simulink model "receiving_app2"  (R2022b)
settings: Solver=FixedStepAuto  StartTime=0.0  StopTime=inf  RelTol=1e-3
libraries: androidcommunicationlib x3, androiduilib x3, androidaudiovideolib x1
settings Model: Creator=Akshat  LastModifiedBy=Akshat
settings OptimizationCC: EnhancedBackFolding=on  PassReuseOutputArgsAs=Individual arguments  ZeroExternalMemoryAtStartup=off  ZeroInternalMemoryAtStartup=off  MaxStackSize=64  OptimizeBlockOrder=speed  DifferentSizesBufferReuse=on  OptimizationCustomize=off  EfficientTunableParamExpr=on
settings DebuggingCC: ParameterTunabilityLossMsg=error
settings HardwareCC: ProdBitPerPointer=32  ProdBitPerSizeT=32  ProdBitPerPtrDiffT=32  ProdLargestAtomicInteger=Long  ProdLargestAtomicFloat=Double  ProdWordSize=32  ProdHWDeviceType=ARM Compatible->ARM Cortex  UseEmbeddedCoderFeatures=off
settings SFSimCC: MATLABDynamicMemAlloc=off
settings RTWCC: Description=Embedded Coder  SystemTargetFile=ert.tlc  HardwareBoard=Android Device  TLCOptions="-aInlineSetEventsForThisBaseRateFcn=TLC_FALSE -aSuppressMultiTaskScheduler=TLC_FALSE  -aRateBasedStepFcn=0"  TemplateMakefile=ert_default_tmf  RTWVerbose=off  Toolchain=Android SDK/NDK Tools
settings CodeAppCC: ForceParamTrailComments=on  IgnoreCustomStorageClasses=off  OperatorAnnotations=on  SimulinkDataObjDesc=on  SFDataObjDesc=on  InsertBlockDesc=on
settings ERTTargetCC: SupportNonInlinedSFcns=on

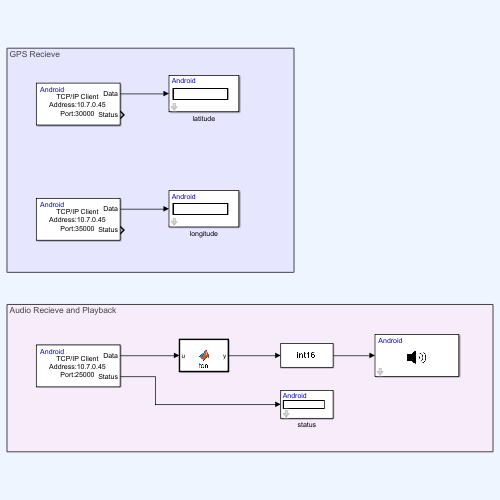
[thumbnail: Simulink's stored preview of the top-level diagram]
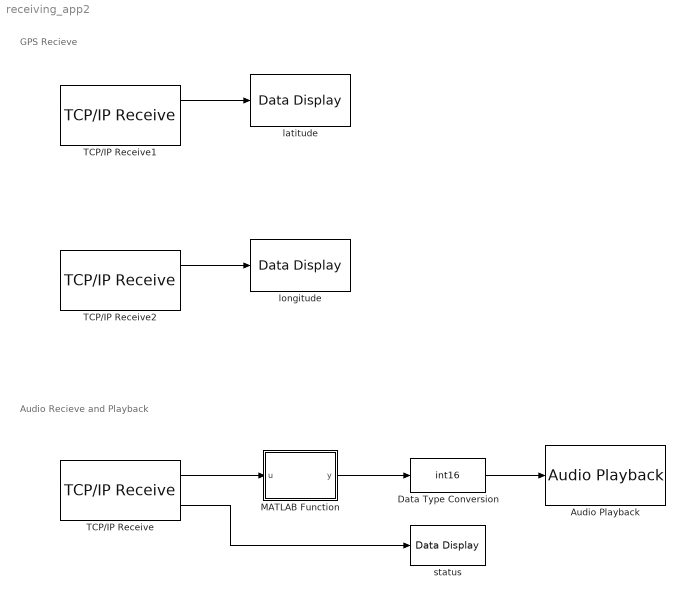
== system receiving_app2 ==
  note: GPS Recieve
  note: Audio Recieve and Playback
  Audio Playback : androidaudiovideolib/Audio Playback  SampleFreq=24000  AudioSamplingFreq=24000  SampleTime=0.1  DeviceStr=0  QueueDuration=0  BlockPlatform=Android
  Data Type Conversion : DataTypeConversion  OutDataTypeStr=int16  SaturateOnIntegerOverflow=off  RndMeth=Floor
  MATLAB Function : MATLAB Function  TreatAsAtomicUnit=on
  TCP/IP Receive : androidcommunicationlib/TCP//IP Receive  TCPReceiveId=receiving_app2/TCP//IP_Receive  Mode_=Client  LocalServerPort_=25000  RemoteAddr_=10.7.0.45  RemoteServerPort_=25000  DataType_=double  DataSize_=300  SampleTime_=0.0125  ClientPortBindingSelection_=off  ClientPortToBind_=35000  BlockingMode_=off  BlockTimeout_=0.1
  TCP/IP Receive1 : androidcommunicationlib/TCP//IP Receive  TCPReceiveId=receiving_app2/TCP//IP_Receive1  Mode_=Client  LocalServerPort_=25000  RemoteAddr_=10.7.0.45  RemoteServerPort_=30000  DataType_=double  DataSize_=1  SampleTime_=0.0125  ClientPortBindingSelection_=off  ClientPortToBind_=35000  BlockingMode_=off  BlockTimeout_=0.1
  TCP/IP Receive2 : androidcommunicationlib/TCP//IP Receive  TCPReceiveId=receiving_app2/TCP//IP_Receive2  Mode_=Client  LocalServerPort_=25000  RemoteAddr_=10.7.0.45  RemoteServerPort_=35000  DataType_=double  DataSize_=1  SampleTime_=0.0125  ClientPortBindingSelection_=off  ClientPortToBind_=35000  BlockingMode_=off  BlockTimeout_=0.1
  latitude : androiduilib/Data Display  DataDisplayId=receiving_app2/latitude  Format=Float  Precision=6  SimulateUsing=Code generation  blockPlatform=Android
  longitude : androiduilib/Data Display  DataDisplayId=receiving_app2/longitude  Format=Float  Precision=6  SimulateUsing=Code generation  blockPlatform=Android
  status : androiduilib/Data Display  DataDisplayId=receiving_app2/status  Format=Float  Precision=6  SimulateUsing=Code generation  blockPlatform=Android
  wires:
  TCP/IP Receive/2 -> status/1
  TCP/IP Receive/1 -> MATLAB Function/1(u)
  MATLAB Function/1(y) -> Data Type Conversion/1
  Data Type Conversion/1 -> Audio Playback/1
  TCP/IP Receive1/1 -> latitude/1
  TCP/IP Receive2/1 -> longitude/1

== matlab function receiving_app2/MATLAB Function ==
  data: u input; y output
function y = fcn(u)

y = [u,u];
